simulink model "EngCylTestNV"  (Simulink 7.5)
settings: Solver=ode45  StartTime=0.0  StopTime=10.0  RelTol=1e-3
values from neighbouring files (symbols this model uses):
  B = [B1;B2]    [GensetRespOptimiztion.m]    (also in GensetRespOptimiztionTorstein.m; Init8RTFLEX68D.m = 0.68; init_MVM.m = 0.127)
  beta = 0.75    [Init8RTFLEX68D.m]
  cAlpha = 1    [Init8RTFLEX68D.m]
  cAStartRef = 104.8    [Init8RTFLEX68D.m]
  cCylHT = [5.3040e-4;-1.1493e0;8.3165e2;-1.9799e5]    [Init8RTFLEX68D.m]
  dCALiftDown = cAVVDownRef(end) - cAVVDownRef(1)    [Init8RTFLEX68D.m]
  dCALiftTopRef = 63.5    [Init8RTFLEX68D.m]
  dCALiftUp = cAVVUpRef(end) - cAVVUpRef(1)    [Init8RTFLEX68D.m]
  Dp = 0.383    [Init8RTFLEX68D.m]
  Ds = 0.079    [Init8RTFLEX68D.m]
  Dv = 0.425    [Init8RTFLEX68D.m]
  ECyl0 = mCyl0.*u    [Init8RTFLEX68D.m]
  fs = 0.0683    [Init8RTFLEX68D.m]    (also in NOxProcessGUI.m = varargin{2}; initHybrid.m; initMV.m; init_MVM.m = 0.0682925799315)
  hn = 42707000    [Init8RTFLEX68D.m]    (also in NOxProcessGUI.m = varargin{3})
  lambdaCrank = 0.5056    [Init8RTFLEX68D.m]
  liftMax = 0.17    [Init8RTFLEX68D.m]
  mbCyl0 = mCyl0.*FCyl0 * fs./(1 + FCyl0*fs)    [Init8RTFLEX68D.m]
  mCp = 10000    [Init8RTFLEX68D.m]
  mCyl0 = pCyl0.*vCyl0 ./ (R.*TCyl0)    [Init8RTFLEX68D.m]
  mqfCycMax = 9.5547e-2    (= 0.095547)    [Init8RTFLEX68D.m]
  nCyl = 8    [Init8RTFLEX68D.m]    (also in init_MVM.m = 6)
  nPort = 28    [Init8RTFLEX68D.m]
  nStroke = 2    [Init8RTFLEX68D.m]
  phi0rad = phi0*pi/180    [Init8RTFLEX68D.m]
  r = 0.035    [Init8RTFLEX68D.m]
  stroke = 2.72    [Init8RTFLEX68D.m]
  vCyl0 = vComp + pi*B^2/4.0*(stroke/2.0*(1.0-cos(phi0rad) +          1.0/lambdaCrank*(1.0-sqrt(1.0 - lambdaCrank^2*sin(phi0rad).^2))))    [Init8RTFLEX68D.m]
  w = 0.021    [Init8RTFLEX68D.m]
  wiebePara = [0.07;0.57;3.05;11;24;56.3;1.5;1;0.7]    [Init8RTFLEX68D.m]
  X = 0.07    [Init8RTFLEX68D.m]
  Y = 0.16    [Init8RTFLEX68D.m]
undefined symbols (not defined in the file or in its folder): cAVVDownRef, cAVVUpRef, liftDownRef, liftUpRef
libraries: EngineSystemSubmodel_SHI x9
settings Model: Creator=KevinKSY  LastModifiedBy=KevinKSY

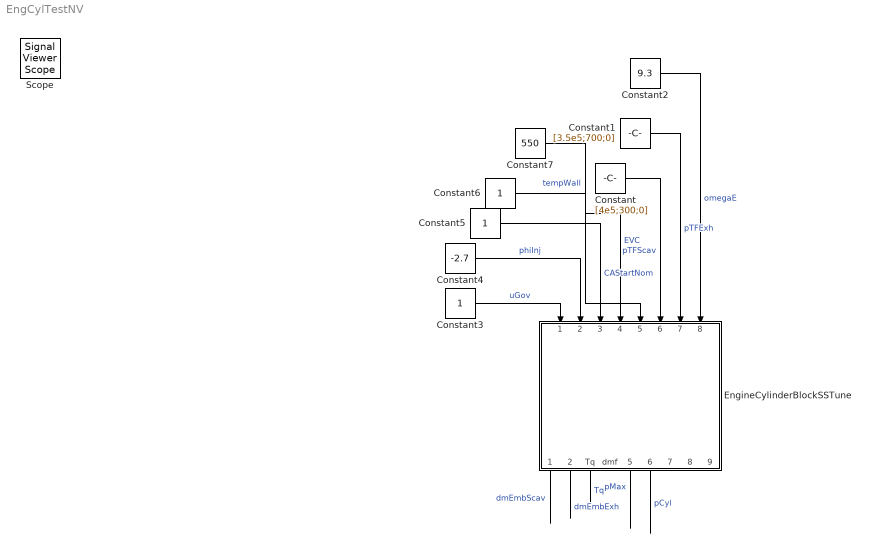
== system EngCylTestNV ==
  Constant : Constant  Value=[4e5;300;0]  OutDataType=fixdt(1, 16)  OutScaling=2^0
  Constant1 : Constant  Value=[3.5e5;700;0]  OutDataType=fixdt(1, 16)  OutScaling=2^0
  Constant2 : Constant  Value=9.3  OutDataType=fixdt(1, 16)  OutScaling=2^0
  Constant3 : Constant  OutDataType=fixdt(1, 16)  OutScaling=2^0
  Constant4 : Constant  Value=-2.7  OutDataType=fixdt(1, 16)  OutScaling=2^0
  Constant5 : Constant  OutDataType=fixdt(1, 16)  OutScaling=2^0
  Constant6 : Constant  OutDataType=fixdt(1, 16)  OutScaling=2^0
  Constant7 : Constant  Value=550  OutDataType=fixdt(1, 16)  OutScaling=2^0
  EngineCylinderBlockSSTune : Subsystem  AncestorBlock=EngineSystemSubmodel_SHI/EngineCylinderBlockSSTune  mask{fs=fs, nStroke=nStroke, hn=hn, nCyl=nCyl, B=B, stroke=stroke, lambdaCrank=lambdaCrank, aCrank=stroke/2, X=X, Y=Y, r=r, nPort=nPort, liftMax=liftMax, Dv=Dv, beta=beta, w=w, Dp=Dp, Ds=Ds, cAVVUpRef=cAVVUpRef, cAVVDownRef=cAVVDownRef, liftUpRef=liftUpRef, liftDownRef=liftDownRef, cAStartRef=cAStartRef, dCALiftUp=dCALiftUp, dCALiftDown=dCALiftDown, dCALiftTopRef=dCALiftTopRef, mCp=mCp, cCylHT=cCylHT, cAlpha=cAlpha, mqfCycMax=mqfCycMax, wiebePara=wiebePara, phi0A=phi0rad, m0A=mCyl0, E0A=ECyl0, mb0A=mbCyl0, V0A=vCyl0}
      mask prompts: fs "Stoichiometric fuel-air ratio"; nStroke "Number of stroke"; hn "Lower heating value of the fuel [J/kg]"; nCyl "Number of cylinders"; B "Bore of the cylinder [m]"; stroke "Stroke [m]"; lambdaCrank "Ratio of length of crank rod to connecting rod"; aCrank "Length of crank rod [m]"; X "Width of inport opening [m]"; Y "Height of inport opening [m]"; r "Raidus of fillet of the opening"; nPort "Number of ports [pcs]"; liftMax "Maximum valve lift [m]"; Dv "Valve head diameter [m]"; beta "Seat angle [rad]"; w "Valve seat width [m]"; Dp "Inner seat diameter [m]"; Ds "Stem diameter [m]"; cAVVUpRef "Crank angle array for opening [deg]"; cAVVDownRef "Crank angle array for closing [deg]"; liftUpRef "Normalized lift array for opening (0~1)"; liftDownRef "Normalized lift array for closing (0~1)"; cAStartRef "Nominal crank angle at start of valve lif [deg]"; dCALiftUp "Nominal duration of crank angle for valve opening [deg]"; dCALiftDown "Nominal duration of crank angle for valve closing [deg]"; dCALiftTopRef "Nominal duration of crank angle for valve open [deg]"; mCp "Heat capacity of the cylinder [J/K]"; cCylHT "Polynomial coefficient for heat rejection model from the cylinder (4 x 1)"; cAlpha "Fitting coefficient for convective heat transfer coefficient"; mqfCycMax "Maximum fuel mass injected per cycle [kg]"; wiebePara "3-Wiebe Parameters (9x1)"; phi0A "Initial crank angle array [deg]"; m0A "Initial mass array [kg]"; E0A "Initial internal energy array [J]"; mb0A "Initial burned fuel mass array [kg]"; V0A "Initial volume array [m3]"
      mask TabNameString: General,General,General,General,Cyl. Dim.,Cyl. Dim.,Cyl. Dim.,Cyl. Dim.,Scav. Port,Scav. Port,Scav. Port,Scav. Port,Exh. VV Dim,Exh. VV Dim,Exh. VV Dim,Exh. VV Dim,Exh. VV Dim,Exh. VV Dim,Exh. VV Profile,Exh. VV Profile,Exh. VV Profile,Exh. VV Profile,Exh. VV Profile,Exh. VV Profile,Exh. VV Profile,Exh. VV Profile,Heat Transfer,Heat Transfer,Heat Transfer,Combustion,Combustion,Initial Conditions,Initial Conditions,Initial Conditions,Initial Conditions,Initial Conditions
  Scope : SignalViewerScope  IOType=viewer  RefreshTime=0.035000
  wires:
  Constant/1 -> EngineCylinderBlockSSTune/6(pTFScav)  "pTFScav"
  Constant1/1 -> EngineCylinderBlockSSTune/7(pTFExh)  "pTFExh"
  Constant2/1 -> EngineCylinderBlockSSTune/8(omega)  "omegaE"
  Constant3/1 -> EngineCylinderBlockSSTune/1(uGov)  "uGov"
  Constant4/1 -> EngineCylinderBlockSSTune/2(phiInj)  "phiInj"
  Constant5/1 -> EngineCylinderBlockSSTune/3(cAStartNom)  "CAStartNom"
  Constant6/1 -> EngineCylinderBlockSSTune/4(dCALiftUp)  "EVC"
  Constant7/1 -> EngineCylinderBlockSSTune/5(tempWall)  "tempWall"
  EngineCylinderBlockSSTune/1(dmEmbScvg) -> ?  "dmEmbScav"
  EngineCylinderBlockSSTune/2(dmEmbExh) -> ?  "dmEmbExh"
  EngineCylinderBlockSSTune/3(Tq) -> ?  "Tq"
  EngineCylinderBlockSSTune/6(pCyl1) -> ?  "pCyl"
  EngineCylinderBlockSSTune/5(pMax) -> ?  "pMax"

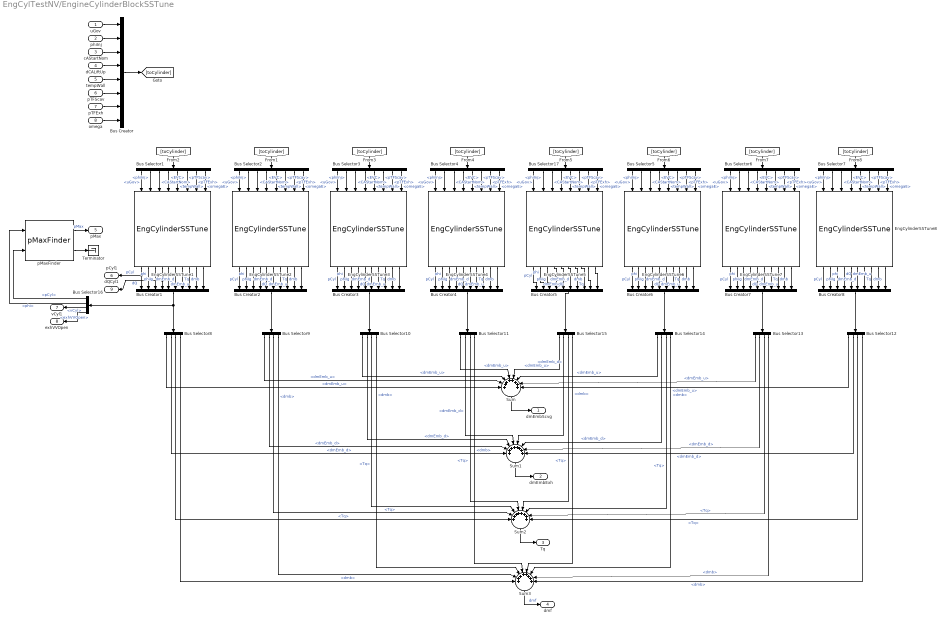
== system EngCylTestNV/EngineCylinderBlockSSTune ==
  uGov : Inport
  phiInj : Inport  Port=2
  cAStartNom : Inport  Port=3
  dCALiftUp : Inport  Port=4
  tempWall : Inport  Port=5
  pTFScav : Inport  Port=6
  pTFExh : Inport  Port=7
  omega : Inport  Port=8
  Bus Creator : BusCreator  Inputs=8
  Bus Creator{1..8} (8 alike) : BusCreator  Inputs=10
  Bus Selector{1..7,17} (8 alike) : BusSelector  OutputSignals=uGov,phiInj,CAStartNom,EVC,tempWall,pTFScav,pTFExh,omegaE
  Bus Selector{8..15} (8 alike) : BusSelector  OutputSignals=dmEmb_u,dmEmb_d,Tq,dmb
  Bus Selector16 : BusSelector  OutputSignals=pCyl,phi,vCyl,exhVVOpen
  EngCylinderSSTune1 : EngineSystemSubmodel_SHI/EngCylinderSSTune  SystemSampleTime=-1  fs=fs  nStroke=nStroke  hn=hn  nCyl=nCyl  iCyl=1  B=B  stroke=stroke  lambdaCrank=lambdaCrank  aCrank=aCrank  X=X  Y=Y  r=r  nPort=nPort  liftMax=liftMax  Dv=Dv  beta=beta  w=w  Dp=Dp  Ds=Ds  cAVVUpRef=cAVVUpRef  cAVVDownRef=cAVVDownRef  liftUpRef=liftUpRef  liftDownRef=liftDownRef  cAStartRef=cAStartRef  dCALiftUp=dCALiftUp  dCALiftDown=dCALiftDown  dCALiftTopRef=dCALiftTopRef  mCp=mCp  cCylHT=cCylHT  cAlpha=cAlpha  mqfCycMax=mqfCycMax  wiebePara=wiebePara  phi0=phi0  m0=mCyl0  E0=ECyl0  mb0=mbCyl0  V0=vCyl0  phi0A=phi0A  m0A=m0A  E0A=E0A  mb0A=mb0A  V0A=V0A
  EngCylinderSSTune{2,5..8} (5 alike) : EngineSystemSubmodel_SHI/EngCylinderSSTune  SystemSampleTime=-1  fs=fs  nStroke=nStroke  hn=hn  nCyl=nCyl  iCyl=2  B=B  stroke=stroke  lambdaCrank=lambdaCrank  aCrank=aCrank  X=X  Y=Y  r=r  nPort=nPort  liftMax=liftMax  Dv=Dv  beta=beta  w=w  Dp=Dp  Ds=Ds  cAVVUpRef=cAVVUpRef  cAVVDownRef=cAVVDownRef  liftUpRef=liftUpRef  liftDownRef=liftDownRef  cAStartRef=cAStartRef  dCALiftUp=dCALiftUp  dCALiftDown=dCALiftDown  dCALiftTopRef=dCALiftTopRef  mCp=mCp  cCylHT=cCylHT  cAlpha=cAlpha  mqfCycMax=mqfCycMax  wiebePara=wiebePara  phi0=phi0  m0=mCyl0  E0=ECyl0  mb0=mbCyl0  V0=vCyl0  phi0A=phi0A  m0A=m0A  E0A=E0A  mb0A=mb0A  V0A=V0A
  EngCylinderSSTune3 : EngineSystemSubmodel_SHI/EngCylinderSSTune  SystemSampleTime=-1  fs=fs  nStroke=nStroke  hn=hn  nCyl=nCyl  iCyl=3  B=B  stroke=stroke  lambdaCrank=lambdaCrank  aCrank=aCrank  X=X  Y=Y  r=r  nPort=nPort  liftMax=liftMax  Dv=Dv  beta=beta  w=w  Dp=Dp  Ds=Ds  cAVVUpRef=cAVVUpRef  cAVVDownRef=cAVVDownRef  liftUpRef=liftUpRef  liftDownRef=liftDownRef  cAStartRef=cAStartRef  dCALiftUp=dCALiftUp  dCALiftDown=dCALiftDown  dCALiftTopRef=dCALiftTopRef  mCp=mCp  cCylHT=cCylHT  cAlpha=cAlpha  mqfCycMax=mqfCycMax  wiebePara=wiebePara  phi0=phi0  m0=mCyl0  E0=ECyl0  mb0=mbCyl0  V0=vCyl0  phi0A=phi0A  m0A=m0A  E0A=E0A  mb0A=mb0A  V0A=V0A
  EngCylinderSSTune4 : EngineSystemSubmodel_SHI/EngCylinderSSTune  SystemSampleTime=-1  fs=fs  nStroke=nStroke  hn=hn  nCyl=nCyl  iCyl=4  B=B  stroke=stroke  lambdaCrank=lambdaCrank  aCrank=aCrank  X=X  Y=Y  r=r  nPort=nPort  liftMax=liftMax  Dv=Dv  beta=beta  w=w  Dp=Dp  Ds=Ds  cAVVUpRef=cAVVUpRef  cAVVDownRef=cAVVDownRef  liftUpRef=liftUpRef  liftDownRef=liftDownRef  cAStartRef=cAStartRef  dCALiftUp=dCALiftUp  dCALiftDown=dCALiftDown  dCALiftTopRef=dCALiftTopRef  mCp=mCp  cCylHT=cCylHT  cAlpha=cAlpha  mqfCycMax=mqfCycMax  wiebePara=wiebePara  phi0=phi0  m0=mCyl0  E0=ECyl0  mb0=mbCyl0  V0=vCyl0  phi0A=phi0A  m0A=m0A  E0A=E0A  mb0A=mb0A  V0A=V0A
  Sum{,1..3} (4 alike) : Sum  Inputs=++++++++  OutDataType=fixdt(1, 16)  OutScaling=2^0
  Terminator : Terminator
  pMaxFinder : EngineSystemSubmodel_SHI/pMaxFinder  SystemSampleTime=-1
  dmEmbScvg : Outport
  dmEmbExh : Outport  Port=2
  Tq : Outport  Port=3
  dmf : Outport  Port=4
  pMax : Outport  Port=5
  pCyl1 : Outport  Port=6
  vCyl1 : Outport  Port=7
  exhVVOpen : Outport  Port=8
  dQCyl1 : Outport  Port=9
  wires:
  Bus Selector16/4 -> exhVVOpen/1  "<exhVVOpen>"
  Bus Selector16/3 -> vCyl1/1  "<vCyl>"
  EngCylinderSSTune8/10 -> Bus Creator8/10
  EngCylinderSSTune8/9 -> Bus Creator8/9
  EngCylinderSSTune7/10 -> Bus Creator7/10
  EngCylinderSSTune7/9 -> Bus Creator7/9
  EngCylinderSSTune6/10 -> Bus Creator6/10
  EngCylinderSSTune6/9 -> Bus Creator6/9
  EngCylinderSSTune4/10 -> Bus Creator4/10
  EngCylinderSSTune4/9 -> Bus Creator4/9
  EngCylinderSSTune3/10 -> Bus Creator3/10
  EngCylinderSSTune3/9 -> Bus Creator3/9
  EngCylinderSSTune2/10 -> Bus Creator2/10
  EngCylinderSSTune2/9 -> Bus Creator2/9
  EngCylinderSSTune1/10 -> Bus Creator1/10
  EngCylinderSSTune1/9 -> Bus Creator1/9
  Bus Selector16/2 -> pMaxFinder/1  "<phi>"
  Bus Selector16/1 -> pMaxFinder/2  "<pCyl>"
  Sum3/1 -> dmf/1  "dmf"
  Bus Selector12/4 -> Sum3/8  "<dmb>"
  Bus Selector13/4 -> Sum3/7  "<dmb>"
  Bus Selector14/4 -> Sum3/6  "<dmb>"
  Bus Selector15/4 -> Sum3/5  "<dmb>"
  Bus Selector11/4 -> Sum3/4  "<dmb>"
  Bus Selector10/4 -> Sum3/3  "<dmb>"
  Bus Selector9/4 -> Sum3/2  "<dmb>"
  Bus Selector8/4 -> Sum3/1  "<dmb>"
  Sum2/1 -> Tq/1
  Bus Selector12/3 -> Sum2/8  "<Tq>"
  Bus Selector13/3 -> Sum2/7  "<Tq>"
  Bus Selector14/3 -> Sum2/6  "<Tq>"
  Bus Selector15/3 -> Sum2/5  "<Tq>"
  Bus Selector11/3 -> Sum2/4  "<Tq>"
  Bus Selector10/3 -> Sum2/3  "<Tq>"
  Bus Selector9/3 -> Sum2/2  "<Tq>"
  Bus Selector8/3 -> Sum2/1  "<Tq>"
  Sum1/1 -> dmEmbExh/1
  Bus Selector12/2 -> Sum1/8  "<dmEmb_d>"
  Bus Selector13/2 -> Sum1/7  "<dmEmb_d>"
  Bus Selector14/2 -> Sum1/6  "<dmEmb_d>"
  Bus Selector15/2 -> Sum1/5  "<dmEmb_d>"
  Bus Selector11/2 -> Sum1/4  "<dmEmb_d>"
  Bus Selector10/2 -> Sum1/3  "<dmEmb_d>"
  Bus Selector9/2 -> Sum1/2  "<dmEmb_d>"
  Bus Selector8/2 -> Sum1/1  "<dmEmb_d>"
  Sum/1 -> dmEmbScvg/1
  Bus Selector12/1 -> Sum/8  "<dmEmb_u>"
  Bus Selector13/1 -> Sum/7  "<dmEmb_u>"
  Bus Selector14/1 -> Sum/6  "<dmEmb_u>"
  Bus Selector15/1 -> Sum/5  "<dmEmb_u>"
  Bus Selector11/1 -> Sum/4  "<dmEmb_u>"
  Bus Selector10/1 -> Sum/3  "<dmEmb_u>"
  Bus Selector9/1 -> Sum/2  "<dmEmb_u>"
  Bus Selector8/1 -> Sum/1  "<dmEmb_u>"
  Bus Creator8/1 -> Bus Selector12/1
  Bus Creator7/1 -> Bus Selector13/1
  Bus Creator6/1 -> Bus Selector14/1
  Bus Creator5/1 -> Bus Selector15/1
  Bus Creator4/1 -> Bus Selector11/1
  Bus Creator3/1 -> Bus Selector10/1
  Bus Creator2/1 -> Bus Selector9/1
  EngCylinderSSTune8/8 -> Bus Creator8/8  "dmb"
  EngCylinderSSTune8/7 -> Bus Creator8/7  "Tq"
  EngCylinderSSTune8/6 -> Bus Creator8/6  "dmEmb_d"
  EngCylinderSSTune8/5 -> Bus Creator8/5  "dmEmb_u"
  EngCylinderSSTune8/4 -> Bus Creator8/4  "dQ"
  EngCylinderSSTune8/3 -> Bus Creator8/3  "phiIg"
  EngCylinderSSTune8/2 -> Bus Creator8/2  "phi"
  EngCylinderSSTune8/1 -> Bus Creator8/1  "pCyl"
  EngCylinderSSTune7/8 -> Bus Creator7/8  "dmb"
  EngCylinderSSTune7/7 -> Bus Creator7/7  "Tq"
  EngCylinderSSTune7/6 -> Bus Creator7/6  "dmEmb_d"
  EngCylinderSSTune7/5 -> Bus Creator7/5  "dmEmb_u"
  EngCylinderSSTune7/4 -> Bus Creator7/4  "dQ"
  EngCylinderSSTune7/3 -> Bus Creator7/3  "phiIg"
  EngCylinderSSTune7/2 -> Bus Creator7/2  "phi"
  EngCylinderSSTune7/1 -> Bus Creator7/1  "pCyl"
  EngCylinderSSTune6/8 -> Bus Creator6/8  "dmb"
  EngCylinderSSTune6/7 -> Bus Creator6/7  "Tq"
  EngCylinderSSTune6/6 -> Bus Creator6/6  "dmEmb_d"
  EngCylinderSSTune6/5 -> Bus Creator6/5  "dmEmb_u"
  EngCylinderSSTune6/4 -> Bus Creator6/4  "dQ"
  EngCylinderSSTune6/3 -> Bus Creator6/3  "phiIg"
  EngCylinderSSTune6/2 -> Bus Creator6/2  "phi"
  EngCylinderSSTune6/1 -> Bus Creator6/1  "pCyl"
  EngCylinderSSTune5/8 -> Bus Creator5/8  "dmb"
  EngCylinderSSTune5/7 -> Bus Creator5/7  "Tq"
  EngCylinderSSTune5/6 -> Bus Creator5/6  "dmEmb_d"
  EngCylinderSSTune5/5 -> Bus Creator5/5  "dmEmb_u"
  EngCylinderSSTune5/4 -> Bus Creator5/4  "dQ"
  EngCylinderSSTune5/3 -> Bus Creator5/3  "phiIg"
  EngCylinderSSTune5/2 -> Bus Creator5/2  "phi"
  EngCylinderSSTune5/1 -> Bus Creator5/1  "pCyl"
  EngCylinderSSTune4/8 -> Bus Creator4/8  "dmb"
  EngCylinderSSTune4/7 -> Bus Creator4/7  "Tq"
  EngCylinderSSTune4/6 -> Bus Creator4/6  "dmEmb_d"
  EngCylinderSSTune4/5 -> Bus Creator4/5  "dmEmb_u"
  EngCylinderSSTune4/4 -> Bus Creator4/4  "dQ"
  EngCylinderSSTune4/3 -> Bus Creator4/3  "phiIg"
  EngCylinderSSTune4/2 -> Bus Creator4/2  "phi"
  EngCylinderSSTune4/1 -> Bus Creator4/1  "pCyl"
  EngCylinderSSTune3/8 -> Bus Creator3/8  "dmb"
  EngCylinderSSTune3/7 -> Bus Creator3/7  "Tq"
  EngCylinderSSTune3/6 -> Bus Creator3/6  "dmEmb_d"
  EngCylinderSSTune3/5 -> Bus Creator3/5  "dmEmb_u"
  EngCylinderSSTune3/4 -> Bus Creator3/4  "dQ"
  EngCylinderSSTune3/3 -> Bus Creator3/3  "phiIg"
  EngCylinderSSTune3/2 -> Bus Creator3/2  "phi"
  EngCylinderSSTune3/1 -> Bus Creator3/1  "pCyl"
  EngCylinderSSTune2/8 -> Bus Creator2/8  "dmb"
  EngCylinderSSTune2/7 -> Bus Creator2/7  "Tq"
  EngCylinderSSTune2/6 -> Bus Creator2/6  "dmEmb_d"
  EngCylinderSSTune2/5 -> Bus Creator2/5  "dmEmb_u"
  EngCylinderSSTune2/4 -> Bus Creator2/4  "dQ"
  EngCylinderSSTune2/3 -> Bus Creator2/3  "phiIg"
  EngCylinderSSTune2/2 -> Bus Creator2/2  "phi"
  EngCylinderSSTune2/1 -> Bus Creator2/1  "pCyl"
  Bus Creator1/1 -> Bus Selector16/1, Bus Selector8/1
  EngCylinderSSTune1/8 -> Bus Creator1/8  "dmb"
  EngCylinderSSTune1/7 -> Bus Creator1/7  "Tq"
  EngCylinderSSTune1/6 -> Bus Creator1/6  "dmEmb_d"
  EngCylinderSSTune1/5 -> Bus Creator1/5  "dmEmb_u"
  EngCylinderSSTune1/4 -> dQCyl1/1, Bus Creator1/4  "dQ"
  EngCylinderSSTune1/3 -> Bus Creator1/3  "phiIg"
  EngCylinderSSTune1/2 -> Bus Creator1/2  "phi"
  EngCylinderSSTune1/1 -> pCyl1/1, Bus Creator1/1  "pCyl"
  [toCylinder] -> Bus Selector7/1
  [toCylinder] -> Bus Selector6/1
  [toCylinder] -> Bus Selector5/1
  [toCylinder] -> Bus Selector17/1
  [toCylinder] -> Bus Selector4/1
  [toCylinder] -> Bus Selector3/1
  [toCylinder] -> Bus Selector1/1
  [toCylinder] -> Bus Selector2/1
  Bus Creator/1 -> [toCylinder]
  omega/1 -> Bus Creator/8
  pTFExh/1 -> Bus Creator/7
  pTFScav/1 -> Bus Creator/6
  tempWall/1 -> Bus Creator/5
  dCALiftUp/1 -> Bus Creator/4
  cAStartNom/1 -> Bus Creator/3
  phiInj/1 -> Bus Creator/2
  uGov/1 -> Bus Creator/1
  pMaxFinder/2 -> Terminator/1
  pMaxFinder/1 -> pMax/1  "pMax"
  Bus Selector7/1 -> EngCylinderSSTune8/1  "<uGov>"
  Bus Selector7/2 -> EngCylinderSSTune8/2  "<phiInj>"
  Bus Selector7/3 -> EngCylinderSSTune8/3  "<CAStartNom>"
  Bus Selector7/4 -> EngCylinderSSTune8/4  "<EVC>"
  Bus Selector7/5 -> EngCylinderSSTune8/5  "<tempWall>"
  Bus Selector7/6 -> EngCylinderSSTune8/6  "<pTFScav>"
  Bus Selector7/7 -> EngCylinderSSTune8/7  "<pTFExh>"
  Bus Selector7/8 -> EngCylinderSSTune8/8  "<omegaE>"
  Bus Selector6/1 -> EngCylinderSSTune7/1  "<uGov>"
  Bus Selector6/2 -> EngCylinderSSTune7/2  "<phiInj>"
  Bus Selector6/3 -> EngCylinderSSTune7/3  "<CAStartNom>"
  Bus Selector6/4 -> EngCylinderSSTune7/4  "<EVC>"
  Bus Selector6/5 -> EngCylinderSSTune7/5  "<tempWall>"
  Bus Selector6/6 -> EngCylinderSSTune7/6  "<pTFScav>"
  Bus Selector6/7 -> EngCylinderSSTune7/7  "<pTFExh>"
  Bus Selector6/8 -> EngCylinderSSTune7/8  "<omegaE>"
  Bus Selector5/1 -> EngCylinderSSTune6/1  "<uGov>"
  Bus Selector5/2 -> EngCylinderSSTune6/2  "<phiInj>"
  Bus Selector5/3 -> EngCylinderSSTune6/3  "<CAStartNom>"
  Bus Selector5/4 -> EngCylinderSSTune6/4  "<EVC>"
  Bus Selector5/5 -> EngCylinderSSTune6/5  "<tempWall>"
  Bus Selector5/6 -> EngCylinderSSTune6/6  "<pTFScav>"
  Bus Selector5/7 -> EngCylinderSSTune6/7  "<pTFExh>"
  Bus Selector5/8 -> EngCylinderSSTune6/8  "<omegaE>"
  Bus Selector1/1 -> EngCylinderSSTune1/1  "<uGov>"
  Bus Selector1/2 -> EngCylinderSSTune1/2  "<phiInj>"
  Bus Selector1/3 -> EngCylinderSSTune1/3  "<CAStartNom>"
  Bus Selector1/4 -> EngCylinderSSTune1/4  "<EVC>"
  Bus Selector1/5 -> EngCylinderSSTune1/5  "<tempWall>"
  Bus Selector1/6 -> EngCylinderSSTune1/6  "<pTFScav>"
  Bus Selector1/7 -> EngCylinderSSTune1/7  "<pTFExh>"
  Bus Selector1/8 -> EngCylinderSSTune1/8  "<omegaE>"
  Bus Selector2/1 -> EngCylinderSSTune2/1  "<uGov>"
  Bus Selector2/2 -> EngCylinderSSTune2/2  "<phiInj>"
  Bus Selector2/3 -> EngCylinderSSTune2/3  "<CAStartNom>"
  Bus Selector2/4 -> EngCylinderSSTune2/4  "<EVC>"
  Bus Selector2/5 -> EngCylinderSSTune2/5  "<tempWall>"
  Bus Selector2/6 -> EngCylinderSSTune2/6  "<pTFScav>"
  Bus Selector2/7 -> EngCylinderSSTune2/7  "<pTFExh>"
  Bus Selector2/8 -> EngCylinderSSTune2/8  "<omegaE>"
  Bus Selector3/1 -> EngCylinderSSTune3/1  "<uGov>"
  Bus Selector3/2 -> EngCylinderSSTune3/2  "<phiInj>"
  Bus Selector3/3 -> EngCylinderSSTune3/3  "<CAStartNom>"
  Bus Selector3/4 -> EngCylinderSSTune3/4  "<EVC>"
  Bus Selector3/5 -> EngCylinderSSTune3/5  "<tempWall>"
  Bus Selector3/6 -> EngCylinderSSTune3/6  "<pTFScav>"
  Bus Selector3/7 -> EngCylinderSSTune3/7  "<pTFExh>"
  Bus Selector3/8 -> EngCylinderSSTune3/8  "<omegaE>"
  Bus Selector4/1 -> EngCylinderSSTune4/1  "<uGov>"
  Bus Selector4/2 -> EngCylinderSSTune4/2  "<phiInj>"
  Bus Selector4/3 -> EngCylinderSSTune4/3  "<CAStartNom>"
  Bus Selector4/4 -> EngCylinderSSTune4/4  "<EVC>"
  Bus Selector4/5 -> EngCylinderSSTune4/5  "<tempWall>"
  Bus Selector4/6 -> EngCylinderSSTune4/6  "<pTFScav>"
  Bus Selector4/7 -> EngCylinderSSTune4/7  "<pTFExh>"
  Bus Selector4/8 -> EngCylinderSSTune4/8  "<omegaE>"
  Bus Selector17/1 -> EngCylinderSSTune5/1  "<uGov>"
  Bus Selector17/2 -> EngCylinderSSTune5/2  "<phiInj>"
  Bus Selector17/3 -> EngCylinderSSTune5/3  "<CAStartNom>"
  Bus Selector17/4 -> EngCylinderSSTune5/4  "<EVC>"
  Bus Selector17/5 -> EngCylinderSSTune5/5  "<tempWall>"
  Bus Selector17/6 -> EngCylinderSSTune5/6  "<pTFScav>"
  Bus Selector17/7 -> EngCylinderSSTune5/7  "<pTFExh>"
  Bus Selector17/8 -> EngCylinderSSTune5/8  "<omegaE>"
  EngCylinderSSTune5/9 -> Bus Creator5/9
  EngCylinderSSTune5/10 -> Bus Creator5/10
